simulink model "Car_smoothmove_testingDec_23_1329_quad"  (Simulink 8.0)
settings: Solver=ode5  StartTime=0.0  StopTime=inf  FixedStep=sample_time  RelTol=1e-3
InitFcn:
  | sample_time=0.005;%0.004;%0.0025;%0.02;
  | sample_time_Vicon = 0.005;
  | DeltaT = 0.02;
  | g = 9.81;
  | H0 = g%0.3165;
  | Kl = 1;
  | 
  | Q6_mass = 0.5;
  | 
  | Q6_Omega_r = 1.5; %for horizon ref
  | Q6_Zeta_r = 0.5; %for horizon ref
  | Q6_Omega_r_h = 2;%for vertical ref
  | Q6_Zeta_r_h = 1; %for vertical ref
  | 
  | 
  | Q6_Omega = 1.5; %for horizon control
  | Q6_Zeta = 0.5; %for horizon control
  | Q6_Omega_h= 2; %for vertical control
  | Q6_Zeta_h = 0.7; %for vertical control
  | 
  | 
  | Q6_acc_max = 5;%horizontal max acc
  | Q6_acc_max_h = 3;%horizontal max acc
  | 
  | omega_circle = 72*pi/180;
  | omega_h = 0.1;%Ascending speed
  | PI = pi;
  | Circle_R = 2.5;
  | MAX_Height = -2;
undefined symbols (not defined in the file): DiscIntNeverNeededParam
libraries: simulink x11, X330_Control x5
(part 2 of 2)

== matlab function UAV 1/Trajectory Logic/Estimation_Subsystem/linear-circular_selector ==
  data: outputx output double; outputy output double; dyaw input double; encir output double; px input double; py input double; enlin output double; st_flag input double
function [outputx,outputy,encir,enlin] = fcn(dyaw,px,py,st_flag)
%#codegen

% select circular or linear estimation in the next sequence
if(st_flag == 0)
if(dyaw>-0.87 && dyaw < 0.87) %define yaw angle in 5 degree as linear motion
    dyaw = 0;
end
if(dyaw == 0)
    enlin = 1;
    encir = 0;
else
    enlin = 0;
    encir = 1;
end
    
else
    enlin = 0;
    encir = 0;
end
outputx = px;
    outputy = py;

== matlab function UAV 1/Trajectory Logic/Estimation_Subsystem/linear_motion_estimation ==
  data: yaw input double; px input double; py input double; estpos output double; enlin input double; estL input double; transveclin output double
function [estpos,transveclin]  = fcn(yaw,px,py,enlin,estL)
%#codegen

%estimate linear motion
if(enlin == 1)
pxy = [px py];
transveclin = [estL * cos(yaw) estL * sin(yaw)];
estpos = pxy + transveclin;
else
    estpos = [0 0];
    transveclin = [0 0];
end

== stateflow chart UAV 1/Trajectory Logic/UAV SF1 ==
  state Landing
    state Decsending
      en:PosDesired = Pos;
      du:PosDesired[2] = (0 - PosDesired[2])*1*DeltaT + PosDesired[2] ;
    state CutThrottle
      du:HoverThrottle = (0.01 - HoverThrottle)*2*DeltaT + HoverThrottle ;
    (default) -> Decsending
    Decsending -> CutThrottle : [Pos[2] > -0.15]
  state Airborne1
    state TakeOff
      du:HoverThrottle = (H0 - HoverThrottle)*2*DeltaT + HoverThrottle ;
    state Hover
      en: PosDesired[2] = -1;
    state capturing_sequence
      state normal_capturing
        en: PosDesired[0] = carest[0]; PosDesired[1] = carest[1]; PosDesired[2] = -0.8
        ex: after(5,sec);
        normal_capturing -> normal_capturing [order 1] : [match_flag==0]
      state success_capturing
        en: PosDesired[0] = Pos[0];PosDesired[1] = Pos[1]; PosDesired[2] = -1.7;
        ex: after(5,sec);
      state capture_landing
        state Decsending1
          en:PosDesired[0] = Pos[0]; PosDesired[1] = Pos[1]; PosDesired[2] = Pos[2]; PosDesired[3] = landing_area[3]
          du:PosDesired[2] = (0 - PosDesired[2])*1*DeltaT + PosDesired[2] ;
        state CutThrottle1
          du:HoverThrottle = (0.01 - HoverThrottle)*2*DeltaT + HoverThrottle ;
        (default) -> Decsending1
        Decsending1 -> CutThrottle1 : [Pos[2] > (landing_area[3]  - 0.2)]
      state Move_to_landing_area
        du: PosDesired[0] = Pos[0]; PosDesired[1] = Pos[1]; PosDesired[2] = -0.8 + landing_area[2];
      state Move_to_landing_area1
        du: PosDesired[0] = landing_area[0]; PosDesired[1] = landing_area[1]; PosDesired[2] = -0.8 + landing_area[2]; PosDesired[3] = landing_area[5]
      success_capturing -> normal_capturing [order 1] : [(car[2] > -0.15)]
      (default) -> normal_capturing
      normal_capturing -> success_capturing [order 1] : [match_flag == 1]
      Move_to_landing_area -> normal_capturing [order 2] : [match_flag==0]
      success_capturing -> Move_to_landing_area [order 2] : [(stable_flag == 1)&(car[2]<-0.15)]
          | {smoothflag == 1;}
      Move_to_landing_area -> Move_to_landing_area [order 3] : [stable_flag == 0]
      Move_to_landing_area -> Move_to_landing_area1 [order 1] : after(10,sec)
      Move_to_landing_area1 -> capture_landing : [stable_flag == 1]
          | {HoverThrottle = 0.01;}
    (default) -> TakeOff : {PosDesired = Pos;  PosDesired[2] = -1;}
    Hover -> capturing_sequence : [RC[5] > 0]
    TakeOff -> Hover : after(5,sec)
        | {PosDesired = Pos;}
    capturing_sequence -> Hover : [RC[5] < 0]
        | {PosDesired = Pos;}
  Landing -> Airborne1 : [RC[6] > 0.5]
  Airborne1 -> Landing : [RC[6] < -0.5]
  (default) -> Landing : {HoverThrottle=0.01;}
  data: PosDesired output double size=4; HoverThrottle output double size=1; Mode output uint8 size=3; RC input double size=8; Pos input double size=4; DeltaT parameter double size=1; H0 parameter double size=1; Kl parameter double size=1; VelCmd local double size=2 =0; line_count local int8 size=1 =0; triangle_count local int8 size=1 =0; T_circle local double size=1; omega_circle parameter double size=1; PI parameter double size=1; omega_h parameter double; Circle_R parameter double size=1; MAX_Height parameter double size=1; carest input double size=2; car input double size=12; landing_area input double size=6; stable_flag input boolean size=1; match_flag input double; smoothflag output boolean size=1 [0..1] =0

== matlab function UAV 1/Trajectory Logic/stable_chk/stablize_checking ==
  data: posx input double; stable_flag output double; posy input double; carx input double; cary input double
function stable_flag = fcn(posx,posy,carx,cary)
%#codegen
subx = abs(posx - carx);
suby = abs(posy - cary);
if(subx < 0.1 && suby < 0.1)
    stable_flag = 1;
else
    stable_flag = 0;
end

== matlab function UAV 1/Trajectory Logic/Subsystem/match_chk ==
  data: vsx input double; match_flag output double; vsy input double
function match_flag = fcn(vsx,vsy)
%#codegen
if(abs(vsx) < 0.2 && abs(vsy) < 0.2)
    match_flag = 1;
else
    match_flag = 0;
end

== stateflow chart UAV 1/Trajectory Logic/UAV SF2 ==
  state Landing
    state Decsending
      en:PosDesired = Pos;
      du:PosDesired[2] = (0 - PosDesired[2])*1*DeltaT + PosDesired[2] ;
    state CutThrottle
      du:HoverThrottle = (0.01 - HoverThrottle)*2*DeltaT + HoverThrottle ;
    (default) -> Decsending
    Decsending -> CutThrottle : [Pos[2] > -0.15]
  state Adjustmenttola
    en: PosDesired[2] = -1; PosDesired[0] = 0; PosDesired[1] =0;
  state Airborne1
    state TakeOff
      du:HoverThrottle = (H0 - HoverThrottle)*2*DeltaT + HoverThrottle ;
    state Hover
      en: PosDesired[2] = -1;
    state capturing_sequence
      state Moving_landing_areaquad1
        du: PosDesired[0] = Pos[0]  + T_line * cos(atan(dx/dy));
        PosDesired[1] = Pos[1] + T_line * sin(atan(dx/dy));
        PosDesired[2] = -1;
        T_line = T_line  + 0.002;
      state increase_height
        en:PosDesired = Pos;
        PosDesired[2] = -1;
      state Hoversequence
        en: PosDesired = Pos; PosDesired[2] = -1;
      state Moving_landing_areaquad2
        du: PosDesired[0] = Pos[0]  + T_line * cos(atan(dx/dy));
        PosDesired[1] = Pos[1] + T_line * sin(atan(dx/dy));
        PosDesired[2] = -1;
        T_line = T_line  + 0.002;
      state Moving_landing_areaquad3
        du: PosDesired[0] = Pos[0]  + T_line * cos(atan(dx/dy) + PI);
        PosDesired[1] = Pos[1] + T_line * sin(atan(dx/dy) + PI);
        PosDesired[2] = -1;
        T_line = T_line  + 0.002;
      state Moving_landing_areaquad4
        du: PosDesired[0] = Pos[0]  + T_line * cos(atan(dx/dy) + PI);
        PosDesired[1] = Pos[1] + T_line * sin(atan(dx/dy) + PI);
        PosDesired[2] = -1;
        T_line = T_line  + 0.002;
      (junction 182) -> increase_height [order 2] : [Pos[0] <-0.01&Pos[0] >0.01 & Pos[1] < -0.01 & Pos[1]>0.01]
          | {T_line = 0.0;}
      (default) -> increase_height : {distanceinitial = distanceLU}
      (junction 181) -> Moving_landing_areaquad4 [order 1] : [quad == 4]
      increase_height -> (junction 181) : [Pos[2] < -0.9 & Pos[2] > -1.1]
          | {T_line = 0.0;}
      (junction 181) -> Moving_landing_areaquad3 [order 2] : [quad == 3]
      (junction 181) -> Moving_landing_areaquad2 [order 3] : [quad == 2]
      (junction 181) -> Moving_landing_areaquad1 [order 4] : [quad == 1]
      Moving_landing_areaquad4 -> (junction 182)
      Moving_landing_areaquad1 -> (junction 182)
      Moving_landing_areaquad3 -> (junction 182)
      Moving_landing_areaquad2 -> (junction 182)
      (junction 182) -> Hoversequence [order 1] : [Pos[0] >=-0.01&Pos[0] <=0.01 & Pos[1] >= -0.01 & Pos[1]<=0.01]
    (default) -> TakeOff : {PosDesired = Pos;  PosDesired[2] = -1;}
    Hover -> capturing_sequence : [RC[5] > 0]
    TakeOff -> Hover : after(5,sec)
        | {PosDesired = Pos;}
    capturing_sequence -> Hover : [RC[5] < 0]
        | {PosDesired = Pos;}
  Landing -> Airborne1 : [RC[6] > 0.5]
  Airborne1 -> Landing : [RC[6] < -0.5]
  (default) -> Landing : {HoverThrottle=0.01;}
  data: PosDesired output double size=4; HoverThrottle output double size=1; Mode output uint8 size=3; RC input double size=8; Pos input double size=4; DeltaT parameter double size=1; H0 parameter double size=1; Kl parameter double size=1; VelCmd local double size=2 =0; line_count local int8 size=1 =0; triangle_count local int8 size=1 =0; T_line local double size=1; omega_circle parameter double size=1; PI parameter double size=1; omega_h parameter double; Circle_R parameter double size=1; MAX_Height parameter double size=1; carest input double size=2; car input double size=12; landing_area input double size=6; stable_flag input boolean size=1; match_flag input double; smoothflag output boolean size=1 [0..1] =0; transvec input double size=2; distanceLU input double size=1; dx input double size=1; dy input double size=1; distanceinitial output double; LAmatch input double size=1; quad input double

== matlab function UAV 1/Trajectory Logic/Dis_calculate ==
  data: landing_areax input double; y output double; landing_areay input double; uavx input double; uavy input double; dx output double; dy output double; quad output double
function [y,dx,dy,quad] = fcn(landing_areax,landing_areay, uavx, uavy)
%#codegen
if(landing_areax>=uavx && landing_areay >= uavy)
    quad = 1;
elseif(landing_areax >=uavx && landing_areay <uavy)
    quad = 2;
elseif(landing_areax < uavx && landing_areay < uavy)
    quad = 3;
elseif(landing_areax < uavx && landing_areay >= uavy)
    quad = 4;
else 
    quad = 0;
end
  dx = landing_areax - uavx;
  dy = landing_areay - uavy;
  y = sqrt(dx^2 + dy^2);

== matlab function UAV 1/Trajectory Logic/matchuav&LA/match_chk ==
  data: vsx input double; match_flag output double; vsy input double
function match_flag = fcn(vsx,vsy)
%#codegen
if(abs(vsx) < 0.1 && abs(vsy) < 0.1)
    match_flag = 1;
else
    match_flag = 0;
end
